simulink model "fixed_wing_sim"  (Simulink 8.7)
settings: Solver=ode4  StartTime=0.0  StopTime=T_sim  FixedStep=ts_sim  MaxStep=10e-3  RelTol=1e-3
InitFcn:
  | % Run the initialization script
  | clear all
  | aerosonde_uav_conf_model
StopFcn:
  | %show_result
  | print_results
values from neighbouring files (symbols this model uses):
  a = param(1)    [get_field.m]    (also in print_results.m = a*scale_fac/1e3; vector_field_parameters.m = 0.85)
  AilBnd = range_ail.*degrees2rad    [aerosonde_uav_conf_model.m]
  aileron_limits = [-20*pi/180;20*pi/180]    [aerosonde_uav_conf_model.m]
  AlphaBnd = range_alpha.*degrees2rad    [aerosonde_uav_conf_model.m]
  amp_theta = amp_theta*2    [vector_field_parameters.m]
  amp_theta_c = ((1/4)*[1 1 1]/6)*U_theta*tau_theta    [vector_field_parameters.m]
  amp_v_c = [1 1 1]*(tau_v*U_v)/6    [vector_field_parameters.m]
  amp_x = [5 5 5]    [vector_field_parameters.m]
  amp_y = [5 5 5]    [vector_field_parameters.m]
  amp_z = amp_z*2    [vector_field_parameters.m]
  amp_z_c = [1 1 1]*(tau_z*U_z)/6/2    [vector_field_parameters.m]
  b = param(2)    [get_field.m]    (also in print_results.m = b*scale_fac/1e3; vector_field_parameters.m = 0.08)
  BetaBnd = range_beta.*degrees2rad    [aerosonde_uav_conf_model.m]
  Bw = 2.8956    [aerosonde_uav_conf_model.m]
  c = param(3)    [get_field.m]    (also in vector_field_parameters.m = -0.13)
  CD_0 = 0.0434    [aerosonde_uav_conf_model.m]
  CD_ail = ones(length(AlphaBnd),1)*CD_aux_ail    [aerosonde_uav_conf_model.m]
  CD_alpha_beta = zeros(length(AlphaBnd),length(BetaBnd))    [aerosonde_uav_conf_model.m]
  CD_elev = ones(length(AlphaBnd),1)*CD_aux_elev    [aerosonde_uav_conf_model.m]
  CD_mind = 0.23    [aerosonde_uav_conf_model.m]
  CD_rud = ones(length(AlphaBnd),1)*CD_aux_rud    [aerosonde_uav_conf_model.m]
  CL_0 = 0.23    [aerosonde_uav_conf_model.m]
  Cl_ail = ones(length(AlphaBnd),1)*Cl_aux_ail    [aerosonde_uav_conf_model.m]
  CL_alpha_beta = CL_alpha*ones(1,length(BetaBnd))    [aerosonde_uav_conf_model.m]
  Cl_alpha_beta = ones(length(AlphaBnd),1)*Cl_beta    [aerosonde_uav_conf_model.m]
  CL_alphadot = 1.9724    [aerosonde_uav_conf_model.m]
  CL_elev = ones(length(AlphaBnd),1)*CL_aux_elev    [aerosonde_uav_conf_model.m]
  Cl_P = ones(length(AlphaBnd),1)*Cl_aux_P    [aerosonde_uav_conf_model.m]
  CL_Q = 7.9543*QBnd    [aerosonde_uav_conf_model.m]
  Cl_R = ones(length(AlphaBnd),1)*Cl_aux_R    [aerosonde_uav_conf_model.m]
  Cl_rud = ones(length(AlphaBnd),1)*Cl_aux_rud    [aerosonde_uav_conf_model.m]
  CLE_alphat = zeros(1,length(AlphaBnd))    [aerosonde_uav_conf_model.m]
  CLE_elev = 0    [aerosonde_uav_conf_model.m]
  Cm0 = 0.135    [aerosonde_uav_conf_model.m]
  Cm_alpha_beta = Cm_alpha*ones(1,length(BetaBnd))    [aerosonde_uav_conf_model.m]
  Cm_alphadot = -10.3796    [aerosonde_uav_conf_model.m]
  Cm_elev = ones(length(AlphaBnd),1)*Cm_aux_elev    [aerosonde_uav_conf_model.m]
  Cm_Q = -38.2067*QBnd    [aerosonde_uav_conf_model.m]
  Cn_ail = ones(length(AlphaBnd),1)*Cn_aux_ail    [aerosonde_uav_conf_model.m]
  Cn_alpha_beta = ones(length(AlphaBnd),1)*Cn_beta    [aerosonde_uav_conf_model.m]
  Cn_P = ones(length(AlphaBnd),1)*Cn_aux_P    [aerosonde_uav_conf_model.m]
  Cn_R = ones(length(AlphaBnd),1)*Cn_aux_R    [aerosonde_uav_conf_model.m]
  Cn_rud = ones(length(AlphaBnd),1)*Cn_aux_rud    [aerosonde_uav_conf_model.m]
  CT_save = CT_save.*10    [aerosonde_uav_conf_model.m]    (also in helice.mat = [0.115262 0.00375054783545 -0.00666475255621 -0.006665219028)
  curve = 1    [vector_field_parameters.m]
  Cw = 0.189941    [aerosonde_uav_conf_model.m]
  CY_ail = ones(length(AlphaBnd),1)*CY_aux_ail    [aerosonde_uav_conf_model.m]
  CY_alpha_beta = ones(length(AlphaBnd),1)*CY_beta    [aerosonde_uav_conf_model.m]
  CY_P = zeros(length(AlphaBnd),length(PBnd))    [aerosonde_uav_conf_model.m]
  CY_R = zeros(length(AlphaBnd),length(RBnd))    [aerosonde_uav_conf_model.m]
  CY_rud = ones(length(AlphaBnd),1)*CY_aux_rud    [aerosonde_uav_conf_model.m]
  d = param(4)    [get_field.m]    (also in vector_field_parameters.m = -0.04)
  D_hel = 0.15    [aerosonde_uav_conf_model.m]
  d_wash = 0    [aerosonde_uav_conf_model.m]
  delta_CD = 1    [aerosonde_uav_conf_model.m]
  delta_CL = 1    [aerosonde_uav_conf_model.m]
  delta_Cl = 1    [aerosonde_uav_conf_model.m]
  delta_Cm = 1    [aerosonde_uav_conf_model.m]
  delta_Cn = 1    [aerosonde_uav_conf_model.m]
  delta_CY = 1    [aerosonde_uav_conf_model.m]
  delta_FT = 1    [aerosonde_uav_conf_model.m]
  Delta_V_EH = [ 2 1.7365 1.2985 1.0890 1.0205]    [aerosonde_uav_conf_model.m]
  Delta_V_J = [ 0 0.4 0.7 1.4 2.1]    [aerosonde_uav_conf_model.m]
  elevator_limits = [-15*pi/180;15*pi/180]    [aerosonde_uav_conf_model.m]
  ElevBnd = range_elev.*degrees2rad    [aerosonde_uav_conf_model.m]
  F_T = 19    [aerosonde_uav_conf_model.m]
  f_theta = ([5 3 1]+rand(1,3))*0.05*2*pi/freq_divisor    [vector_field_parameters.m]
  f_theta_c = ([5 3 1]+rand(1,3))*0.05*2*pi/freq_divisor    [vector_field_parameters.m]
  f_v_c = ([4 2 0.5]+rand(1,3))*0.05*2*pi/freq_divisor    [vector_field_parameters.m]
  f_x = ([6 4 2]+rand(1,3))*0.05*2*pi/freq_divisor    [vector_field_parameters.m]
  f_y = ([6 4 2]+rand(1,3))*0.05*2*pi/freq_divisor    [vector_field_parameters.m]
  f_z = ([6 4 2]+rand(1,3))*0.05*2*pi/freq_divisor    [vector_field_parameters.m]
  f_z_c = ([4 2 0.5]+rand(1,3))*0.05*2*pi/freq_divisor    [vector_field_parameters.m]
  g1 = param(5)    [get_field.m]    (also in vector_field_parameters.m = 4)
  gain_G = param(6)    [get_field.m]    (also in vector_field_parameters.m = 2.5)
  gravity = 9.807    [aerosonde_uav_conf_model.m]
  H_0 = 200    [vector_field_parameters.m]
  Heq = 200    [aerosonde_uav_conf_model.m]    (also in vector_field_parameters.m)
  induced_drag = 1/(pi*AR*osw)    (= 0.0278403324809)    [aerosonde_uav_conf_model.m]
  isTrimming = 0    [aerosonde_uav_conf_model.m]
  J_save = J_save.*1.5    [aerosonde_uav_conf_model.m]    (also in helice.mat = [0 1.22229381539 1.27367709689 1.27367940534 1.27361400442 1)
  Jx = 0.7795    [aerosonde_uav_conf_model.m]
  Jxz = 0.1211    [aerosonde_uav_conf_model.m]
  Jy = 1.122    [aerosonde_uav_conf_model.m]
  Jz = 1.752    [aerosonde_uav_conf_model.m]
  KC_h = 0.28    [aerosonde_uav_conf_model.m]
  KC_phi = -1.18    [aerosonde_uav_conf_model.m]
  KC_psi = 0.03    [aerosonde_uav_conf_model.m]
  KC_r = -0.0073    [aerosonde_uav_conf_model.m]
  KC_theta = -1.1482    [aerosonde_uav_conf_model.m]
  KC_vt = 0.9948*1    (= 0.9948)    [aerosonde_uav_conf_model.m]
  KE = -0.1562    [aerosonde_uav_conf_model.m]
  Kp = 0.18    [vector_field_parameters.m]
  KR = 0.0130    (= 0.013)    [aerosonde_uav_conf_model.m]
  Ksad = param(3)    [get_field.m]    (also in print_results.m = Ksad*scale_fac/1e3; vector_field_parameters.m = 0)
  KT = 0.0792    [aerosonde_uav_conf_model.m]
  Kv = 1    [vector_field_parameters.m]
  LIM_CENTER = LIM_CENTER*scale_fac/1e3    [print_results.m]    (also in vector_field_parameters.m = 0.2)
  M = 8.5    [aerosonde_uav_conf_model.m]    (also in print_results.m = 0)
  motor_min = 0.1    [aerosonde_uav_conf_model.m]
  motor_rate = 1    [aerosonde_uav_conf_model.m]
  p_theta = rand(1,3)*2*pi    [vector_field_parameters.m]
  p_theta_c = rand(1,3)*2*pi    [vector_field_parameters.m]
  p_v_c = rand(1,3)*2*pi    [vector_field_parameters.m]
  p_x = rand(1,3)*2*pi    [vector_field_parameters.m]
  p_y = rand(1,3)*2*pi    [vector_field_parameters.m]
  p_z = rand(1,3)*2*pi    [vector_field_parameters.m]
  p_z_c = rand(1,3)*2*pi    [vector_field_parameters.m]
  PBnd = range_P.*degrees2rad    [aerosonde_uav_conf_model.m]
  perc_int_max = 0.8    [aerosonde_uav_conf_model.m]
  phi_max = 20*pi/180    (= 0.349065850399)    [aerosonde_uav_conf_model.m]
  phi_min = -20*pi/180    (= -0.349065850399)    [aerosonde_uav_conf_model.m]
  QBnd = range_Q.*degrees2rad    [aerosonde_uav_conf_model.m]
  r = sqrt(m)    [animation.m]    (also in print_results.m)
  r_aero_abc = r_aero_struct*[-1 0 0;0 1 0;0 0 -1]    [aerosonde_uav_conf_model.m]
  r_cg_abc = r_cg_struct*[-1 0 0;0 1 0;0 0 -1]    [aerosonde_uav_conf_model.m]
  r_motor_abc = r_motor_struct*[-1 0 0;0 1 0;0 0 -1]    [aerosonde_uav_conf_model.m]
  r_tail_abc = r_aero_struct*[-1 0 0;0 1 0;0 0 -1]    [aerosonde_uav_conf_model.m]
  RBnd = range_R.*degrees2rad    [aerosonde_uav_conf_model.m]
  rho = 0.1    [aerosonde_uav_conf_model.m]
  ... (+40 more)
undefined symbols (not defined in the file or in its folder): Earth, F, Light, MIL, WGS84
libraries: aerolibwind2 x2, aerolibtransform2 x2, aerolibfltsims x1, aerolibconvert2 x1, dspsigops x1
(part 1 of 3)
settings Model: Creator=torres  LastModifiedBy=adrianomcr  SimulationMode=accelerator
settings DataIOCC: SignalLoggingSaveFormat=ModelDataLogs  InspectSignalLogs=on
settings OptimizationCC: ExpressionDepthLimit=2147483647  EfficientMapNaN2IntZero=off
settings DebuggingCC: SolverPrmCheckMsg=warning  FcnCallInpInsideContextMsg=UseLocalSettings  UnconnectedInputMsg=none  UnconnectedOutputMsg=none  StateNameClashWarn=warning
settings HardwareCC: TargetBitPerLong=64  TargetBitPerPointer=64  TargetLongLongMode=on  TargetIntDivRoundTo=Zero  TargetEndianess=LittleEndian  TargetWordSize=64  TargetHWDeviceType=MATLAB Host  ProdEqTarget=off
settings SFSimCC: SimParseCustomCode=off
settings CodeAppCC: MaxIdLength=128
settings GRTTargetCC: GeneratePreprocessorConditionals=Use local settings  CombineOutputUpdateFcns=off  GRTInterface=on
settings ConfigComp: CovSFcnEnable=off

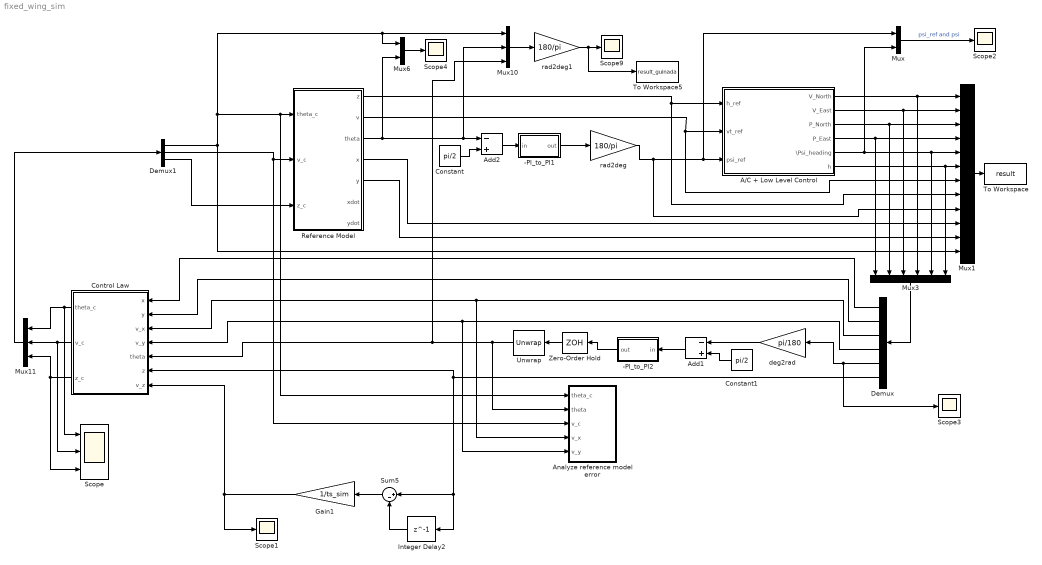
== system fixed_wing_sim ==
  -PI_to_PI1 : Subsystem
      mask Display: disp('-pi to pi')
  -PI_to_PI2 : Subsystem
      mask Display: disp('-pi to pi')
  "A/C + Low Level Control " : Subsystem
  Add1 : Sum  Inputs=-+
  Add2 : Sum  Inputs=-+
  Analyze reference model error : Subsystem
  Constant : Constant  Value=pi/2
  Constant1 : Constant  Value=pi/2
  Control Law : Subsystem
  Demux : Demux  Outputs=6
  Demux1 : Demux  Outputs=3
  Gain1 : Gain  Gain=1/ts_sim
  Integer Delay2 : Delay  DelayLength=1  InitialCondition=H_0  InputProcessing=Inherited
  Mux : Mux  Inputs=2
  Mux1 : Mux  Inputs=12
  Mux10 : Mux  Inputs=3
  Mux11 : Mux  Inputs=3
  Mux3 : Mux  Inputs=6
  Mux6 : Mux  Inputs=2
  Reference Model : Subsystem
  Scope : Scope  NumInputPorts=3
  Scope{1..4,9} (5 alike) : Scope
  Sum5 : Sum  Inputs=|+-
  To Workspace : ToWorkspace  VariableName=result  SaveFormat=Structure With Time  SampleTime=-1
  To Workspace5 : ToWorkspace  VariableName=result_guinada  SaveFormat=Structure With Time  SampleTime=-1
  Unwrap : dspsigops/Unwrap  tol=pi  InputProcessing=Inherited (this choice will be removed - see release notes)  running=off
  Zero-Order Hold : ZeroOrderHold  SampleTime=ts_sim
  deg2rad : Gain  Gain=pi/180
  rad2deg : Gain  Gain=180/pi
  rad2deg1 : Gain  Gain=180/pi
  wires:
  Add2/1 -> -PI_to_PI1/1(in)
  "A/C + Low Level Control "/5(\Psi_heading) -> Mux1/5, Mux3/5, Mux/2
  Reference Model/2(v) -> "A/C + Low Level Control "/2(vt_ref), Mux1/7
  Mux/1 -> Scope2/1  "psi_ref and psi"
  Reference Model/1(z) -> Mux1/8, "A/C + Low Level Control "/1(h_ref)
  -PI_to_PI1/1(out) -> rad2deg/1
  rad2deg/1 -> Mux/1, "A/C + Low Level Control "/3(psi_ref), Mux1/9
  Mux1/1 -> To Workspace/1
  "A/C + Low Level Control "/1(V_North) -> Mux1/1, Mux3/4
  "A/C + Low Level Control "/2(V_East) -> Mux1/2, Mux3/3
  "A/C + Low Level Control "/3(P_North) -> Mux1/3, Mux3/2
  "A/C + Low Level Control "/4(P_East) -> Mux1/4, Mux3/1
  "A/C + Low Level Control "/6(h) -> Mux3/6, Mux1/6
  Add1/1 -> -PI_to_PI2/1(in)
  Constant1/1 -> Add1/2
  deg2rad/1 -> Add1/1
  Demux/3 -> Analyze reference model error/4(v_x), Control Law/3(v_x)
  Mux3/1 -> Demux/1
  Mux6/1 -> Scope4/1
  Demux/5 -> Scope3/1, deg2rad/1
  Demux/1 -> Control Law/1(x)
  Demux/2 -> Control Law/2(y)
  Zero-Order Hold/1 -> Unwrap/1
  -PI_to_PI2/1(out) -> Zero-Order Hold/1
  Mux10/1 -> rad2deg1/1
  Reference Model/3(theta) -> Mux6/2, Mux10/2, Add2/1
  Mux11/1 -> Demux1/1
  Demux1/2 -> Analyze reference model error/3(v_c), Reference Model/2(v_c)
  Demux1/1 -> Mux1/12, Analyze reference model error/1(theta_c), Reference Model/1(theta_c), Mux10/1, Mux6/1
  Constant/1 -> Add2/2
  rad2deg1/1 -> To Workspace5/1, Scope9/1
  Demux/4 -> Analyze reference model error/5(v_y), Control Law/4(v_y)
  Reference Model/4(x) -> Mux1/10
  Reference Model/5(y) -> Mux1/11
  Demux1/3 -> Reference Model/3(z_c)
  Demux/6 -> Integer Delay2/1, Sum5/1, Control Law/6(z)
  Sum5/1 -> Gain1/1
  Gain1/1 -> Scope1/1, Control Law/7(v_z)
  Integer Delay2/1 -> Sum5/2
  Control Law/1(theta_c) -> Scope/1, Mux11/1
  Control Law/2(v_c) -> Scope/2, Mux11/2
  Control Law/3(z_c) -> Mux11/3, Scope/3
  Unwrap/1 -> Analyze reference model error/2(theta), Control Law/5(theta), Mux10/3

== system fixed_wing_sim/-PI_to_PI1 ==
  in : Inport
  Constant : Constant  Value=pi
  Fcn : Fcn  Expr=atan2(sin(u),cos(u))
  Gain : Gain  Gain=2
  Math Function : Math  Operator=mod  SaturateOnIntegerOverflow=on
  Sum : Sum  Inputs=|++
  Sum1 : Sum  Inputs=|+-
  out : Outport
  wires:
  Constant/1 -> Sum/2, Gain/1, Sum1/2
  Sum/1 -> Math Function/1
  Gain/1 -> Math Function/2
  Math Function/1 -> Sum1/1
  in/1 -> Fcn/1
  Fcn/1 -> out/1

== system fixed_wing_sim/-PI_to_PI2 ==
  in : Inport
  Constant : Constant  Value=pi
  Fcn : Fcn  Expr=atan2(sin(u),cos(u))
  Gain : Gain  Gain=2
  Math Function : Math  Operator=mod  SaturateOnIntegerOverflow=on
  Sum : Sum  Inputs=|++
  Sum1 : Sum  Inputs=|+-
  out : Outport
  wires:
  Constant/1 -> Sum/2, Gain/1, Sum1/2
  Sum/1 -> Math Function/1
  Gain/1 -> Math Function/2
  Math Function/1 -> Sum1/1
  in/1 -> Fcn/1
  Fcn/1 -> out/1

== system fixed_wing_sim/A/C + Low Level Control  ==
  h_ref : Inport
  vt_ref : Inport  Port=2
  psi_ref : Inport  Port=3
  -180_to_180 : Subsystem
      mask Display: disp('-180 to +180')
  Abs : Abs
  Add1 : Sum  Inputs=+-
  Add4 : Sum  Inputs=-+
  Gain : Gain  Gain=KE
  Gain1 : Gain  Gain=KT
  PID h : Subsystem
  PID psi (modified) : Subsystem
  UAV Internal Closed Loops : Subsystem
  V_North : Outport
  V_East : Outport  Port=2
  P_North : Outport  Port=3
  P_East : Outport  Port=4
  \Psi_heading : Outport  Port=5
  h : Outport  Port=6
  wires:
  PID h/1(theta_ref) -> UAV Internal Closed Loops/1(ref_theta)
  Add4/1 -> PID h/1(erro), Gain1/1
  PID psi (modified)/1(phi_ref) -> Abs/1, UAV Internal Closed Loops/2(ref_phi)
  Gain1/1 -> UAV Internal Closed Loops/3(uk_thro)
  Add1/1 -> -180_to_180/1(in)
  Gain/1 -> UAV Internal Closed Loops/4(uk_elev)
  UAV Internal Closed Loops/4(\Psi_heading) -> Add1/2, \Psi_heading/1
  Abs/1 -> Gain/1
  UAV Internal Closed Loops/3(h) -> Add4/1, h/1
  h_ref/1 -> Add4/2
  psi_ref/1 -> Add1/1
  vt_ref/1 -> UAV Internal Closed Loops/5(ref_vt)
  UAV Internal Closed Loops/1(V_North) -> V_North/1
  UAV Internal Closed Loops/5(P_North) -> P_North/1
  UAV Internal Closed Loops/6(P_East) -> P_East/1
  UAV Internal Closed Loops/2(V_East) -> V_East/1
  -180_to_180/1(out) -> PID psi (modified)/1(erro)

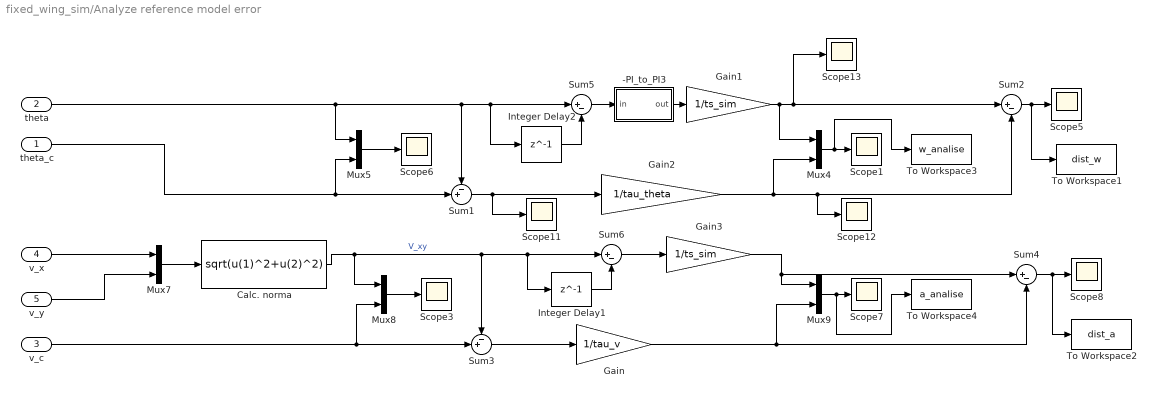
== system fixed_wing_sim/Analyze reference model error ==
  theta_c : Inport
  theta : Inport  Port=2
  v_c : Inport  Port=3
  v_x : Inport  Port=4
  v_y : Inport  Port=5
  -PI_to_PI3 : Subsystem
      mask Display: disp('-pi to pi')
  Calc. norma : Fcn  Expr=sqrt(u(1)^2+u(2)^2)
  Gain : Gain  Gain=1/tau_v
  Gain1 : Gain  Gain=1/ts_sim
  Gain2 : Gain  Gain=1/tau_theta
  Gain3 : Gain  Gain=1/ts_sim
  Integer Delay1 : Delay  DelayLength=1  InitialCondition=Veq  InputProcessing=Inherited
  Integer Delay2 : Delay  DelayLength=1  InitialCondition=theta_0  InputProcessing=Inherited
  Mux{4..5,7..9} (5 alike) : Mux  Inputs=2
  Scope{1,3,5..8,11..13} (9 alike) : Scope
  Sum1 : Sum  Inputs=-+|
  Sum{2,4..6} (4 alike) : Sum  Inputs=|+-
  Sum3 : Sum  Inputs=-+|
  To Workspace1 : ToWorkspace  VariableName=dist_w  SaveFormat=Structure With Time  SampleTime=-1
  To Workspace2 : ToWorkspace  VariableName=dist_a  SaveFormat=Structure With Time  SampleTime=-1
  To Workspace3 : ToWorkspace  VariableName=w_analise  SaveFormat=Structure With Time  SampleTime=-1
  To Workspace4 : ToWorkspace  VariableName=a_analise  SaveFormat=Structure With Time  SampleTime=-1
  wires:
  Sum2/1 -> To Workspace1/1, Scope5/1
  Mux5/1 -> Scope6/1
  Gain2/1 -> Mux4/2, Scope12/1, Sum2/2
  Calc. norma/1 -> Mux8/1, Sum3/1, Integer Delay1/1, Sum6/1  "V_xy"
  Mux8/1 -> Scope3/1
  Sum3/1 -> Gain/1
  Mux9/1 -> To Workspace4/1, Scope7/1
  Gain/1 -> Sum4/2, Mux9/2
  Sum4/1 -> To Workspace2/1, Scope8/1
  Integer Delay2/1 -> Sum5/2
  Gain1/1 -> Scope13/1, Sum2/1, Mux4/1
  Mux4/1 -> To Workspace3/1, Scope1/1
  Integer Delay1/1 -> Sum6/2
  Sum6/1 -> Gain3/1
  Gain3/1 -> Sum4/1, Mux9/1
  Sum1/1 -> Scope11/1, Gain2/1
  Sum5/1 -> -PI_to_PI3/1(in)
  -PI_to_PI3/1(out) -> Gain1/1
  Mux7/1 -> Calc. norma/1
  v_x/1 -> Mux7/1
  v_y/1 -> Mux7/2
  v_c/1 -> Sum3/2, Mux8/2
  theta_c/1 -> Mux5/2, Sum1/2
  theta/1 -> Mux5/1, Integer Delay2/1, Sum5/1, Sum1/1

== system fixed_wing_sim/Control Law ==
  x : Inport
  y : Inport  Port=2
  v_x : Inport  Port=3
  v_y : Inport  Port=4
  theta : Inport  Port=5
  z : Inport  Port=6
  v_z : Inport  Port=7
  Actuation Error : Subsystem
  Control law : MATLAB Function  TreatAsAtomicUnit=on
  Demux : Demux  Outputs=9
  Measurement Error : Subsystem
  Mux14 : Mux  Inputs=2
  Potental functions : Scope  NumInputPorts=2
  Potental functions1 : Scope  NumInputPorts=9
  Sum{,1..2,5} (4 alike) : Sum  Inputs=|++
  Sum3 : Sum  Inputs=++|
  Sum4 : Sum  Inputs=++|
  Sum6 : Sum  Inputs=++|
  To Workspace6 : ToWorkspace  VariableName=PotFncs  SaveFormat=Structure With Time  SampleTime=-1
  theta_c : Outport
  v_c : Outport  Port=2
  z_c : Outport  Port=3
  wires:
  v_x/1 -> Control law/3(xd)
  v_y/1 -> Control law/4(yd)
  Mux14/1 -> To Workspace6/1
  Control law/4(V_theta) -> Potental functions/1, Mux14/1
  Control law/5(V_fld) -> Potental functions/2, Mux14/2
  Sum/1 -> Control law/1(x)
  x/1 -> Sum/1
  Measurement Error/2(Noise_x) -> Sum/2
  Sum1/1 -> Control law/2(y)
  y/1 -> Sum1/1
  Measurement Error/3(Noise_y) -> Sum1/2
  Sum2/1 -> Control law/5(theta)
  Control law/1(theta_c) -> Sum3/2
  Sum3/1 -> theta_c/1
  Sum4/1 -> v_c/1
  Control law/2(v_c) -> Sum4/2
  Actuation Error/2(Noise_v_c) -> Sum4/1
  Actuation Error/1(Noise_theta_c) -> Sum3/1
  theta/1 -> Sum2/1
  Measurement Error/1(Noise_theta) -> Sum2/2
  v_z/1 -> Control law/7(zd)
  Sum5/1 -> Control law/6(z)
  z/1 -> Sum5/1
  Measurement Error/4(Noise_z) -> Sum5/2
  Sum6/1 -> z_c/1
  Control law/3(z_c) -> Sum6/2
  Actuation Error/3(Noise_z_c) -> Sum6/1
  Control law/6(teste) -> Demux/1
  Demux/1 -> Potental functions1/1
  Demux/2 -> Potental functions1/2
  Demux/9 -> Potental functions1/9
  Demux/8 -> Potental functions1/8
  Demux/7 -> Potental functions1/7
  Demux/6 -> Potental functions1/6
  Demux/5 -> Potental functions1/5
  Demux/4 -> Potental functions1/4
  Demux/3 -> Potental functions1/3

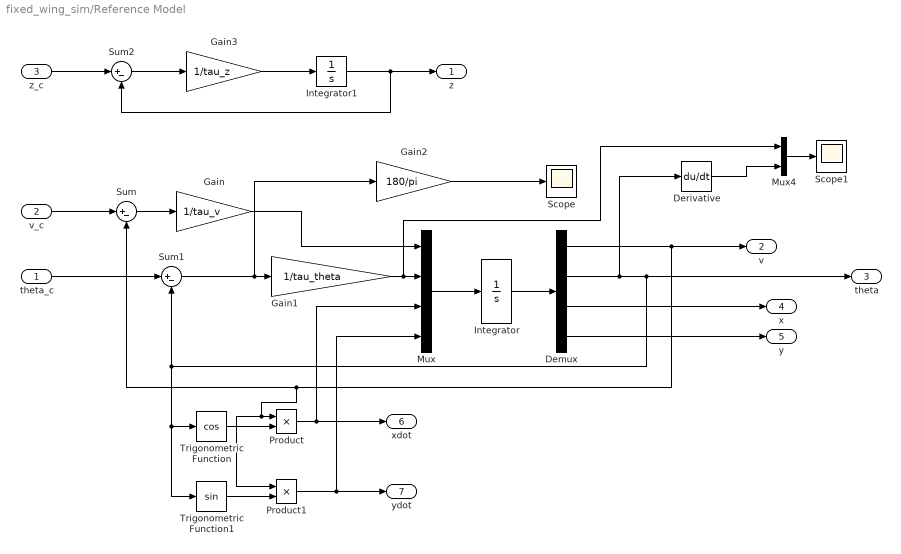
== system fixed_wing_sim/Reference Model ==
  theta_c : Inport
  v_c : Inport  Port=2
  z_c : Inport  Port=3
  Demux : Demux
  Derivative : Derivative
  Gain : Gain  Gain=1/tau_v
  Gain1 : Gain  Gain=1/tau_theta
  Gain2 : Gain  Gain=180/pi
  Gain3 : Gain  Gain=1/tau_z
  Integrator : Integrator  InitialCondition=x0_refmodel
  Integrator1 : Integrator  InitialCondition=H_0
  Mux : Mux
  Mux4 : Mux  Inputs=2
  Product : Product  RndMeth=Zero
  Product1 : Product  RndMeth=Zero
  Scope : Scope
  Scope1 : Scope
  Sum : Sum  Inputs=|+-
  Sum1 : Sum  Inputs=|+-
  Sum2 : Sum  Inputs=|+-
  Trigonometric Function : Trigonometry  Operator=cos
  Trigonometric Function1 : Trigonometry
  z : Outport
  v : Outport  Port=2
  theta : Outport  Port=3
  x : Outport  Port=4
  y : Outport  Port=5
  xdot : Outport  Port=6
  ydot : Outport  Port=7
  wires:
  v_c/1 -> Sum/1
  Sum/1 -> Gain/1
  Gain/1 -> Mux/1
  Sum1/1 -> Gain1/1, Gain2/1
  Gain1/1 -> Mux4/1, Mux/2
  theta_c/1 -> Sum1/1
  Mux/1 -> Integrator/1
  Integrator/1 -> Demux/1
  Demux/1 -> v/1, Product1/1, Product/1, Sum/2
  Demux/2 -> Derivative/1, theta/1, Trigonometric Function/1, Trigonometric Function1/1, Sum1/2
  Trigonometric Function/1 -> Product/2
  Trigonometric Function1/1 -> Product1/2
  Product/1 -> Mux/3, xdot/1
  Product1/1 -> Mux/4, ydot/1
  Demux/3 -> x/1
  Demux/4 -> y/1
  Gain2/1 -> Scope/1
  Mux4/1 -> Scope1/1
  Derivative/1 -> Mux4/2
  z_c/1 -> Sum2/1
  Sum2/1 -> Gain3/1
  Gain3/1 -> Integrator1/1
  Integrator1/1 -> Sum2/2, z/1

== system fixed_wing_sim/A/C + Low Level Control /-180_to_180 ==
  in : Inport
  Constant : Constant  Value=pi
  Gain : Gain  Gain=2
  Math Function : Math  Operator=mod  SaturateOnIntegerOverflow=on
  Sum : Sum  Inputs=|++
  Sum1 : Sum  Inputs=|+-
  deg2rad : Gain  Gain=pi/180
  rad2deg : Gain  Gain=180/pi
  out : Outport
  wires:
  Constant/1 -> Sum/2, Gain/1, Sum1/2
  in/1 -> deg2rad/1
  Sum/1 -> Math Function/1
  Gain/1 -> Math Function/2
  Math Function/1 -> Sum1/1
  Sum1/1 -> rad2deg/1
  rad2deg/1 -> out/1
  deg2rad/1 -> Sum/1

== system fixed_wing_sim/A/C + Low Level Control /PID h ==
  erro : Inport
  Add : Sum  Inputs=+-++
  Constant : Constant  Value=TI_h
  Divide : Product  Inputs=*/
  Gain : Gain  Gain=KC_h
  Gain1 : Gain
  Gain2 : Gain  Gain=1/rho
  Integrator : Integrator  InitialCondition=x0_uav(5)  LimitOutput=on  UpperSaturationLimit=perc_int_max*theta_max  LowerSaturationLimit=perc_int_max*theta_min
  Rate Limiter1 : RateLimiter  RisingSlewLimit=theta_rate  FallingSlewLimit=-theta_rate
  Saturation1 : Saturate  UpperLimit=theta_max  LowerLimit=theta_min
  Transfer Fcn : TransferFcn  Numerator=[1/rho]  Denominator=[rho*TD_h 1]
  theta_ref : Outport
  wires:
  Add/1 -> Rate Limiter1/1
  Transfer Fcn/1 -> Add/2
  Integrator/1 -> Add/4
  Divide/1 -> Integrator/1
  Constant/1 -> Divide/2
  Gain1/1 -> Add/1
  Gain2/1 -> Add/3
  erro/1 -> Gain/1
  Gain/1 -> Gain1/1, Transfer Fcn/1, Gain2/1, Divide/1
  Rate Limiter1/1 -> Saturation1/1
  Saturation1/1 -> theta_ref/1

== system fixed_wing_sim/A/C + Low Level Control /PID psi (modified) ==
  erro : Inport
  Add : Sum  Inputs=+-++
  Constant : Constant  Value=TI_psi
  Divide : Product  Inputs=*/
  Gain : Gain  Gain=KC_psi
  Gain1 : Gain
  Gain2 : Gain  Gain=1/rho
  Integrator : Integrator  LimitOutput=on  UpperSaturationLimit=phi_max  LowerSaturationLimit=phi_min
  Rate Limiter2 : RateLimiter  RisingSlewLimit=roll_rate  FallingSlewLimit=-roll_rate
  Saturation2 : Saturate  UpperLimit=phi_max  LowerLimit=phi_min
  Transfer Fcn : TransferFcn  Numerator=[1/rho]  Denominator=[rho*TD_psi 1]
  phi_ref : Outport
  wires:
  Transfer Fcn/1 -> Add/2
  Gain1/1 -> Add/1
  Gain2/1 -> Add/3
  erro/1 -> Gain/1
  Gain/1 -> Gain1/1, Transfer Fcn/1, Gain2/1, Divide/1
  Rate Limiter2/1 -> Saturation2/1
  Saturation2/1 -> phi_ref/1
  Add/1 -> Rate Limiter2/1
  Integrator/1 -> Add/4
  Divide/1 -> Integrator/1
  Constant/1 -> Divide/2

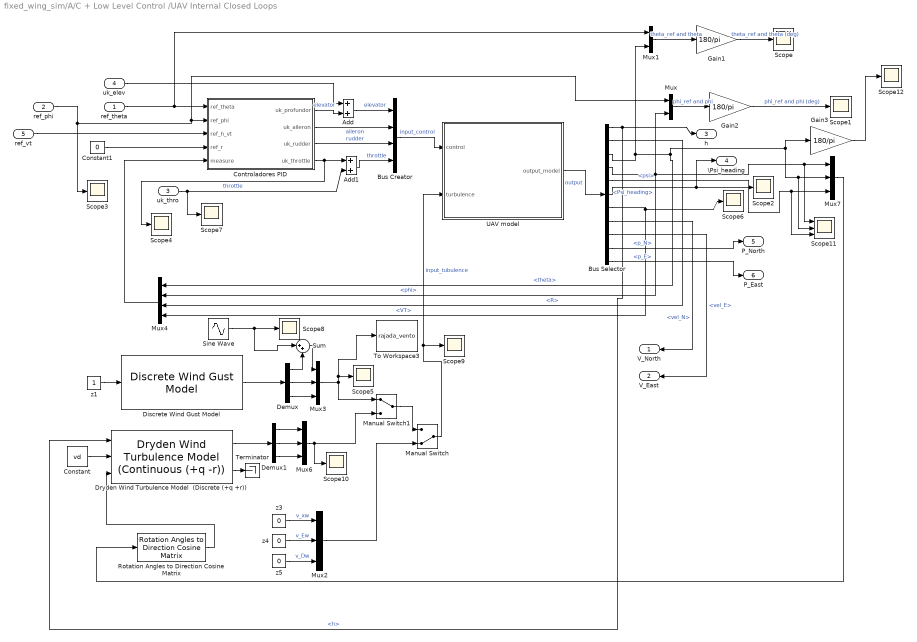
== system fixed_wing_sim/A/C + Low Level Control /UAV Internal Closed Loops ==
  ref_theta : Inport
  ref_phi : Inport  Port=2
  uk_thro : Inport  Port=3
  uk_elev : Inport  Port=4
  ref_vt : Inport  Port=5
  Add : Sum
  Add1 : Sum
  Bus Creator : BusCreator  Inputs=4
  Bus Selector : BusSelector  OutputSignals=h,R,theta,phi,psi,Psi_heading,VT,vel_N,vel_E,p_N,p_E
  Constant : Constant  Value=vd
  Constant1 : Constant  Value=0
  Controladores PID : Subsystem
  Demux : Demux  Outputs=3
  Demux1 : Demux  Outputs=3
  Discrete Wind Gust Model : aerolibwind2/Discrete Wind Gust Model  units=Metric (MKS)  Gx=on  Gy=on  Gz=on  t_0=0  d_m=[20 20 20]  v_m=[5.75 0 0]
  Dryden Wind Turbulence Model  (Discrete (+q +r)) : aerolibwind2/Dryden Wind Turbulence Model  (Continuous (+q -r))  units=Metric (MKS)  spec=MIL-F-8785C  model=Continuous Dryden (+q +r)  W20=1  Wdeg=0  TurbProb=10^-2 - Light  L_high=533.4  Wingspan=Bw  ts=ts_sim  Seed=[23341 23342 23343 23344]  T_on=on
  Gain1 : Gain  Gain=180/pi
  Gain2 : Gain  Gain=180/pi
  Gain3 : Gain  Gain=180/pi
  Manual Switch : ManualSwitch  CurrentSetting=0
  Manual Switch1 : ManualSwitch
  Mux : Mux  Inputs=2
  Mux1 : Mux  Inputs=2
  Mux{2..3,6..7} (4 alike) : Mux  Inputs=3
  Mux4 : Mux
  Rotation Angles to Direction Cosine Matrix : aerolibtransform2/Rotation Angles to Direction Cosine Matrix  rotationOrder=ZYX
  Scope{,1..10,12} (12 alike) : Scope
  Scope11 : Scope  NumInputPorts=3
  Sine Wave : Sin  Amplitude=2  Frequency=0.1  SampleTime=0
  Sum : Sum  Inputs=|++
  Terminator : Terminator
  To Workspace3 : ToWorkspace  VariableName=rajada_vento  SaveFormat=Structure With Time  SampleTime=-1
  UAV model : Subsystem
      mask Display: image(imread('Figures/rascal.jpg'))
  z1 : Constant
  z3 : Constant  Value=0
  z4 : Constant  Value=0
  z5 : Constant  Value=0
  V_North : Outport
  V_East : Outport  Port=2
  h : Outport  Port=3
  \Psi_heading : Outport  Port=4
  P_North : Outport  Port=5
  P_East : Outport  Port=6
  wires:
  Controladores PID/3(uk_rudder) -> Bus Creator/3  "rudder"
  UAV model/1(output_model) -> Bus Selector/1  "output"
  Bus Creator/1 -> UAV model/1(control)  "input_control"
  Manual Switch/1 -> UAV model/2(turbulence), Scope9/1  "input_tubulence"
  z4/1 -> Mux2/2  "v_Ew"
  z5/1 -> Mux2/3  "v_Dw"
  Mux4/1 -> Controladores PID/5(measure)
  Bus Selector/7 -> Scope6/1, Mux4/4  "<VT>"
  Controladores PID/2(uk_aileron) -> Bus Creator/2  "aileron"
  Bus Selector/2 -> Mux4/3  "<R>"
  ref_theta/1 -> Controladores PID/1(ref_theta), Mux1/1
  ref_phi/1 -> Controladores PID/2(ref_phi), Mux/1, Scope3/1
  Constant1/1 -> Controladores PID/4(ref_r)
  Controladores PID/4(uk_throttle) -> Scope4/1, Add1/1  "throttle"
  Add1/1 -> Bus Creator/4  "throttle"
  uk_thro/1 -> Scope7/1, Add1/2
  Controladores PID/1(uk_profundor) -> Add/2  "elevator"
  Add/1 -> Bus Creator/1  "elevator"
  uk_elev/1 -> Add/1
  Mux1/1 -> Gain1/1  "theta_ref and theta"
  Mux/1 -> Gain2/1  "phi_ref and phi"
  ref_vt/1 -> Controladores PID/3(ref_h_vt)
  Bus Selector/8 -> V_North/1  "<vel_N>"
  Bus Selector/9 -> V_East/1  "<vel_E>"
  Bus Selector/10 -> P_North/1  "<p_N>"
  Bus Selector/11 -> P_East/1  "<p_E>"
  Bus Selector/1 -> Dryden Wind Turbulence Model  (Discrete (+q +r))/1, h/1  "<h>"
  Bus Selector/6 -> Scope2/1, \Psi_heading/1  "<Psi_heading>"
  Bus Selector/4 -> Mux4/2, Scope11/1, Mux7/1, Mux/2  "<phi>"
  Bus Selector/3 -> Mux4/1, Scope11/2, Mux7/2, Gain3/1, Mux1/2  "<theta>"
  Gain1/1 -> Scope/1  "theta_ref and theta (deg)"
  Gain2/1 -> Scope1/1  "phi_ref and phi (deg)"
  z1/1 -> Discrete Wind Gust Model/1
  z3/1 -> Mux2/1  "v_xw"
  Mux2/1 -> Manual Switch/2
  Discrete Wind Gust Model/1 -> Demux/1
  Demux/2 -> Mux3/2
  Demux/3 -> Mux3/3
  Mux3/1 -> To Workspace3/1, Scope5/1, Manual Switch1/1
  Demux1/2 -> Mux6/2
  Demux1/3 -> Mux6/3
  Demux1/1 -> Mux6/1
  Mux6/1 -> Manual Switch1/2, Scope10/1
  Dryden Wind Turbulence Model  (Discrete (+q +r))/2 -> Terminator/1
  Rotation Angles to Direction Cosine Matrix/1 -> Dryden Wind Turbulence Model  (Discrete (+q +r))/3
  Mux7/1 -> Rotation Angles to Direction Cosine Matrix/1
  Bus Selector/5 -> Scope11/3, Mux7/3  "<psi>"
  Constant/1 -> Dryden Wind Turbulence Model  (Discrete (+q +r))/2
  Manual Switch1/1 -> Manual Switch/1
  Dryden Wind Turbulence Model  (Discrete (+q +r))/1 -> Demux1/1
  Sine Wave/1 -> Scope8/1, Sum/1
  Demux/1 -> Sum/2
  Sum/1 -> Mux3/1
  Gain3/1 -> Scope12/1

== system fixed_wing_sim/Analyze reference model error/-PI_to_PI3 ==
  in : Inport
  Constant : Constant  Value=pi
  Fcn : Fcn  Expr=atan2(sin(u),cos(u))
  Gain : Gain  Gain=2
  Math Function : Math  Operator=mod  SaturateOnIntegerOverflow=on
  Sum : Sum  Inputs=|++
  Sum1 : Sum  Inputs=|+-
  out : Outport
  wires:
  Constant/1 -> Sum/2, Gain/1, Sum1/2
  Sum/1 -> Math Function/1
  Gain/1 -> Math Function/2
  Math Function/1 -> Sum1/1
  in/1 -> Fcn/1
  Fcn/1 -> out/1

== system fixed_wing_sim/Control Law/Actuation Error ==
  note: Disturbance in the theta_c control signal
  note: Disturbance in the v_c control signal
  note: Disturbance in the z_c control signal
  Constant : Constant  Value=0.0001
  Constant1 : Constant  Value=0.0001
  Constant2 : Constant  Value=0.0001
  Demux : Demux  Outputs=3
  Gain : Gain
  Gain1 : Gain  Gain=0.8
  Gain2 : Gain  Gain=0.001
  Manual Switch Noise : ManualSwitch
  Mux1 : Mux  Inputs=3
  Mux14 : Mux  Inputs=3
  Scope : Scope  NumInputPorts=3
  Sine Wave : Sin  Amplitude=amp_theta_c(1)  Frequency=f_theta_c(1)  Phase=p_theta_c(1)  SampleTime=0
  Sine Wave1 : Sin  Amplitude=amp_theta_c(2)  Frequency=f_theta_c(2)  Phase=p_theta_c(2)  SampleTime=0
  Sine Wave2 : Sin  Amplitude=amp_theta_c(3)  Frequency=f_theta_c(3)  Phase=p_theta_c(3)  SampleTime=0
  Sine Wave3 : Sin  Amplitude=amp_v_c(1)  Frequency=f_v_c(1)  Phase=p_v_c(1)  SampleTime=0
  Sine Wave4 : Sin  Amplitude=amp_v_c(2)  Frequency=f_v_c(2)  Phase=p_v_c(2)  SampleTime=0
  Sine Wave5 : Sin  Amplitude=amp_v_c(3)  Frequency=f_v_c(3)  Phase=p_v_c(3)  SampleTime=0
  Sine Wave6 : Sin  Amplitude=amp_z_c(1)  Frequency=f_z_c(1)  Phase=p_z_c(1)  SampleTime=0
  Sine Wave7 : Sin  Amplitude=amp_z_c(2)  Frequency=f_z_c(2)  Phase=p_z_c(2)  SampleTime=0
  Sine Wave8 : Sin  Amplitude=amp_z_c(3)  Frequency=f_z_c(3)  Phase=p_z_c(3)  SampleTime=0
  Sum : Sum  Inputs=+++
  Sum1 : Sum  Inputs=+++
  Sum2 : Sum  Inputs=+++
  Noise_theta_c : Outport
  Noise_v_c : Outport  Port=2
  Noise_z_c : Outport  Port=3
  wires:
  Sine Wave1/1 -> Sum/2
  Sine Wave/1 -> Sum/1
  Sine Wave2/1 -> Sum/3
  Sine Wave4/1 -> Sum1/2
  Sine Wave3/1 -> Sum1/1
  Sine Wave5/1 -> Sum1/3
  Sum/1 -> Scope/1, Mux14/1  "Noise theta_c"
  Sum1/1 -> Gain/1
  Constant1/1 -> Mux1/2
  Constant/1 -> Mux1/1
  Mux14/1 -> Manual Switch Noise/1
  Mux1/1 -> Gain2/1
  Manual Switch Noise/1 -> Gain1/1
  Demux/2 -> Noise_v_c/1
  Demux/1 -> Noise_theta_c/1
  Gain/1 -> Scope/2, Mux14/2  "Noise v_c"
  Sine Wave7/1 -> Sum2/2
  Sine Wave6/1 -> Sum2/1
  Sine Wave8/1 -> Sum2/3
  Constant2/1 -> Mux1/3
  Sum2/1 -> Scope/3, Mux14/3  "Noise z_c"
  Demux/3 -> Noise_z_c/1
  Gain1/1 -> Demux/1
  Gain2/1 -> Manual Switch Noise/2

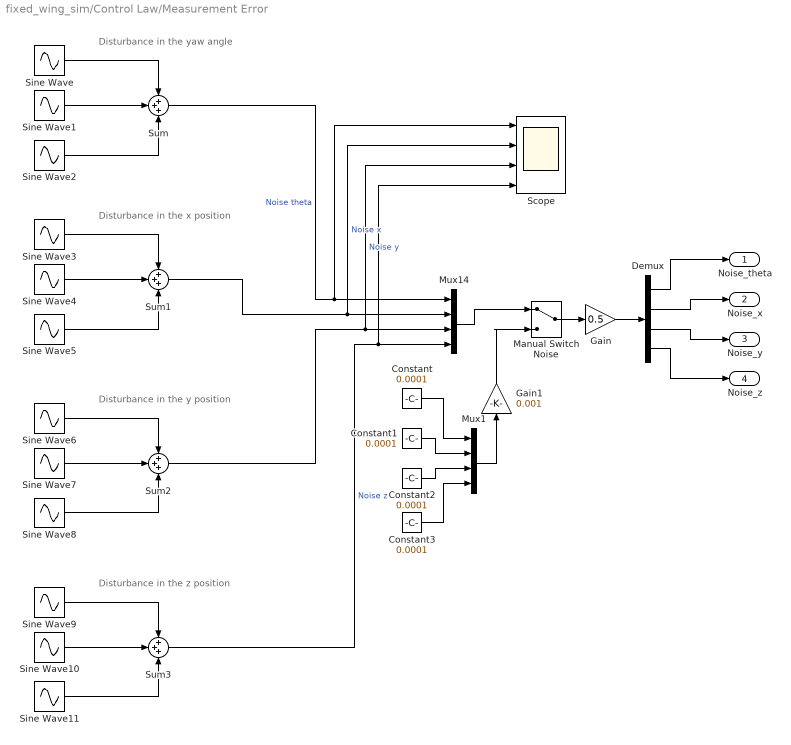
== system fixed_wing_sim/Control Law/Measurement Error ==
  note: Disturbance in the yaw angle
  note: Disturbance in the x position
  note: Disturbance in the y position
  note: Disturbance in the z position
  Constant{,1..3} (4 alike) : Constant  Value=0.0001
  Demux : Demux
  Gain : Gain  Gain=0.5
  Gain1 : Gain  Gain=0.001
  Manual Switch Noise : ManualSwitch
  Mux1 : Mux
  Mux14 : Mux
  Scope : Scope  NumInputPorts=4
  Sine Wave : Sin  Amplitude=amp_theta(1)  Frequency=f_theta(1)  Phase=p_theta(1)  SampleTime=0
  Sine Wave1 : Sin  Amplitude=amp_theta(2)  Frequency=f_theta(2)  Phase=p_theta(2)  SampleTime=0
  Sine Wave10 : Sin  Amplitude=amp_z(2)  Frequency=f_z(2)  Phase=p_z(2)  SampleTime=0
  Sine Wave11 : Sin  Amplitude=amp_z(3)  Frequency=f_z(3)  Phase=p_z(3)  SampleTime=0
  Sine Wave2 : Sin  Amplitude=amp_theta(3)  Frequency=f_theta(3)  Phase=p_theta(3)  SampleTime=0
  Sine Wave3 : Sin  Amplitude=amp_x(1)  Frequency=f_x(1)  Phase=p_x(1)  SampleTime=0
  Sine Wave4 : Sin  Amplitude=amp_x(2)  Frequency=f_x(2)  Phase=p_x(2)  SampleTime=0
  Sine Wave5 : Sin  Amplitude=amp_x(3)  Frequency=f_x(3)  Phase=p_x(3)  SampleTime=0
  Sine Wave6 : Sin  Amplitude=amp_y(1)  Frequency=f_y(1)  Phase=p_y(1)  SampleTime=0
  Sine Wave7 : Sin  Amplitude=amp_y(2)  Frequency=f_y(2)  Phase=p_y(2)  SampleTime=0
  Sine Wave8 : Sin  Amplitude=amp_y(3)  Frequency=f_y(3)  Phase=p_y(3)  SampleTime=0
  Sine Wave9 : Sin  Amplitude=amp_z(1)  Frequency=f_z(1)  Phase=p_z(1)  SampleTime=0
  Sum{,1..3} (4 alike) : Sum  Inputs=+++
  Noise_theta : Outport
  Noise_x : Outport  Port=2
  Noise_y : Outport  Port=3
  Noise_z : Outport  Port=4
  wires:
  Sine Wave1/1 -> Sum/2
  Sine Wave/1 -> Sum/1
  Sine Wave2/1 -> Sum/3
  Sine Wave4/1 -> Sum1/2
  Sine Wave3/1 -> Sum1/1
  Sine Wave5/1 -> Sum1/3
  Sine Wave7/1 -> Sum2/2
  Sine Wave6/1 -> Sum2/1
  Sine Wave8/1 -> Sum2/3
  Sum/1 -> Scope/1, Mux14/1  "Noise theta"
  Sum1/1 -> Scope/2, Mux14/2  "Noise x"
  Sum2/1 -> Scope/3, Mux14/3  "Noise y"
  Mux14/1 -> Manual Switch Noise/1
  Mux1/1 -> Gain1/1
  Manual Switch Noise/1 -> Gain/1
  Demux/2 -> Noise_x/1
  Demux/1 -> Noise_theta/1
  Demux/3 -> Noise_y/1
  Sine Wave10/1 -> Sum3/2
  Sine Wave9/1 -> Sum3/1
  Sine Wave11/1 -> Sum3/3
  Sum3/1 -> Scope/4, Mux14/4  "Noise z"
  Demux/4 -> Noise_z/1
  Constant1/1 -> Mux1/2
  Constant/1 -> Mux1/1
  Constant2/1 -> Mux1/3
  Constant3/1 -> Mux1/4
  Gain/1 -> Demux/1
  Gain1/1 -> Manual Switch Noise/2

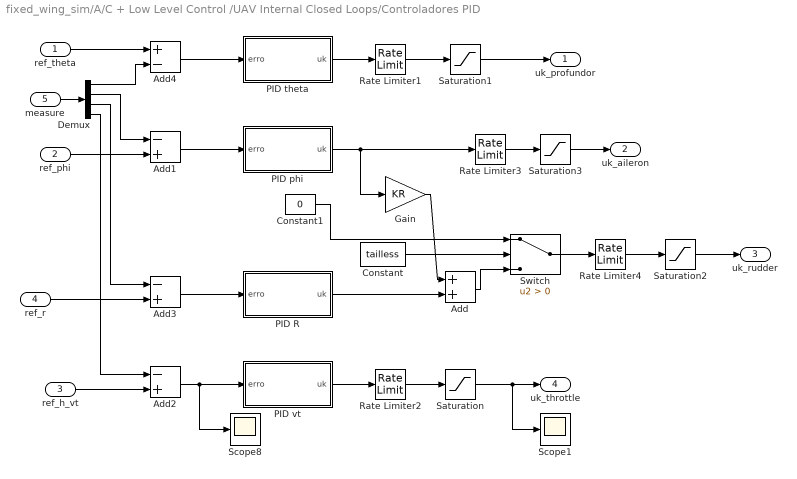
== system fixed_wing_sim/A/C + Low Level Control /UAV Internal Closed Loops/Controladores PID ==
  ref_theta : Inport
  ref_phi : Inport  Port=2
  ref_h_vt : Inport  Port=3
  ref_r : Inport  Port=4
  measure : Inport  Port=5
  Add : Sum
  Add1 : Sum  Inputs=-+
  Add2 : Sum  Inputs=-+
  Add3 : Sum  Inputs=-+
  Add4 : Sum  Inputs=+-
  Constant : Constant  Value=tailless
  Constant1 : Constant  Value=0
  Demux : Demux
  Gain : Gain  Gain=KR
  PID R : Subsystem
  PID phi : Subsystem
  PID theta : Subsystem
  PID vt : Subsystem
  Rate Limiter1 : RateLimiter  RisingSlewLimit=servo_rate  FallingSlewLimit=-servo_rate
  Rate Limiter2 : RateLimiter  RisingSlewLimit=motor_rate  FallingSlewLimit=-motor_rate
  Rate Limiter3 : RateLimiter  RisingSlewLimit=servo_rate  FallingSlewLimit=-servo_rate
  Rate Limiter4 : RateLimiter  RisingSlewLimit=servo_rate  FallingSlewLimit=-servo_rate
  Saturation : Saturate  UpperLimit=1  LowerLimit=motor_min
  Saturation1 : Saturate  UpperLimit=elevator_limits(2)  LowerLimit=elevator_limits(1)
  Saturation2 : Saturate  UpperLimit=rudder_limits(2)  LowerLimit=rudder_limits(1)
  Saturation3 : Saturate  UpperLimit=aileron_limits(2)  LowerLimit=aileron_limits(1)
  Scope1 : Scope
  Scope8 : Scope
  Switch : Switch  Criteria=u2 > Threshold
  uk_profundor : Outport
  uk_aileron : Outport  Port=2
  uk_rudder : Outport  Port=3
  uk_throttle : Outport  Port=4
  wires:
  ref_theta/1 -> Add4/1
  Add4/1 -> PID theta/1(erro)
  measure/1 -> Demux/1
  Demux/1 -> Add4/2
  PID theta/1(uk) -> Rate Limiter1/1
  Rate Limiter1/1 -> Saturation1/1
  PID vt/1(uk) -> Rate Limiter2/1
  Rate Limiter2/1 -> Saturation/1
  Add2/1 -> Scope8/1, PID vt/1(erro)
  PID phi/1(uk) -> Rate Limiter3/1, Gain/1
  Rate Limiter3/1 -> Saturation3/1
  Add1/1 -> PID phi/1(erro)
  ref_phi/1 -> Add1/2
  ref_h_vt/1 -> Add2/2
  Constant/1 -> Switch/2
  Rate Limiter4/1 -> Saturation2/1
  Constant1/1 -> Switch/1
  Demux/2 -> Add1/1
  Demux/3 -> Add3/1
  Demux/4 -> Add2/1
  Add3/1 -> PID R/1(erro)
  Switch/1 -> Rate Limiter4/1
  Add/1 -> Switch/3
  Gain/1 -> Add/1
  PID R/1(uk) -> Add/2
  ref_r/1 -> Add3/2
  Saturation1/1 -> uk_profundor/1
  Saturation3/1 -> uk_aileron/1
  Saturation2/1 -> uk_rudder/1
  Saturation/1 -> Scope1/1, uk_throttle/1

== system fixed_wing_sim/A/C + Low Level Control /UAV Internal Closed Loops/UAV model ==
  control : Inport
  turbulence : Inport  Port=2
  Aerodynamics Equations : Subsystem
      mask Display: image(imread('Figures/aerod.jpg'))
  Atmosphere Model : Subsystem
      mask Display: image(imread('Figures/atmosphere.jpg'))
  Body-Axes 6DOF Equations : Subsystem
      mask Display: image(imread('Figures/forces1.jpg'))
  Constant : Constant  Value=gravity
  Motor Equations : Subsystem
      mask Display: image(imread('Figures/motor_G26.jpg'))
  Output : Subsystem
  Scope2 : Scope
  Servos : Subsystem
      mask Display: image(imread('Figures/servo1.jpg'))
  To Workspace3 : ToWorkspace  VariableName=comando_motor  SaveFormat=Structure With Time  SampleTime=-1
  rpm : Terminator
  output_model : Outport
  wires:
  Body-Axes 6DOF Equations/1(var_states) -> Output/1(states), Aerodynamics Equations/1(var_states), Atmosphere Model/1(var_states)
  Aerodynamics Equations/1(F_Aero_ABC) -> Body-Axes 6DOF Equations/1(F_Aero_ABC)  "Fa_ABC"
  Servos/1(angle_servos) -> Aerodynamics Equations/3(servos)  "command_servos"
  Body-Axes 6DOF Equations/2(acc_x_y_z) -> Output/2(acc)  "acc"
  Aerodynamics Equations/4(V_wind) -> Output/3(V_WIND), Motor Equations/1(Airspeed)  "V_WIND"
  Output/1(Out_model) -> output_model/1
  Constant/1 -> Atmosphere Model/2(gravity)
  Atmosphere Model/1(atmosphere) -> Aerodynamics Equations/2(atmosphere), Motor Equations/2(Atmosphere)
  Aerodynamics Equations/3(F_Tail_ABC) -> Body-Axes 6DOF Equations/3(F_tail_ABC)  "F_tail_ABC"
  Motor Equations/1(F_Thrust_ABC) -> Body-Axes 6DOF Equations/4(F_Thrust_ABC)  "F_Thrust"
  Aerodynamics Equations/2(M_Aero_ABC) -> Body-Axes 6DOF Equations/2(M_Aero_ABC)  "Ma_ABC"
  Servos/2(th_servo) -> Scope2/1, To Workspace3/1, Motor Equations/3(throttle)  "throttle 0% a 100%"
  Motor Equations/2(Delta_V_EH) -> Aerodynamics Equations/4(Delta_V_EH)  "Delta_V_EH"
  turbulence/1 -> Body-Axes 6DOF Equations/5(turb_NED)
  control/1 -> Servos/1(control)
  Body-Axes 6DOF Equations/3(v_ABC') -> Aerodynamics Equations/5(v_ABC')
  Body-Axes 6DOF Equations/4(V_NED) -> Output/4(V_NED)
  Motor Equations/3(RPM) -> rpm/1

== system fixed_wing_sim/A/C + Low Level Control /UAV Internal Closed Loops/Controladores PID/PID R ==
  erro : Inport
  Add : Sum  Inputs=+-++
  Constant : Constant  Value=TI_r
  Divide : Product  Inputs=*/
  Gain : Gain  Gain=KC_r
  Gain1 : Gain
  Gain2 : Gain  Gain=1/rho
  Integrator : Integrator  InitialCondition=u0_uav(3)  LimitOutput=on  UpperSaturationLimit=perc_int_max*rudder_limits(2)  LowerSaturationLimit=-perc_int_max*rudder_limits(2)
  Transfer Fcn : TransferFcn  Numerator=[1/rho]  Denominator=[rho*TD_r 1]
  uk : Outport
  wires:
  Add/1 -> uk/1
  Transfer Fcn/1 -> Add/2
  Integrator/1 -> Add/4
  Divide/1 -> Integrator/1
  Constant/1 -> Divide/2
  Gain1/1 -> Add/1
  Gain2/1 -> Add/3
  erro/1 -> Gain/1
  Gain/1 -> Gain1/1, Transfer Fcn/1, Gain2/1, Divide/1

== system fixed_wing_sim/A/C + Low Level Control /UAV Internal Closed Loops/Controladores PID/PID phi ==
  erro : Inport
  Add : Sum  Inputs=+-++
  Constant : Constant  Value=TI_phi
  Divide : Product  Inputs=*/
  Gain : Gain  Gain=KC_phi
  Gain1 : Gain
  Gain2 : Gain  Gain=1/rho
  Integrator : Integrator  InitialCondition=u0_uav(2)  LimitOutput=on  UpperSaturationLimit=perc_int_max*aileron_limits(2)  LowerSaturationLimit=-perc_int_max*aileron_limits(2)
  Transfer Fcn : TransferFcn  Numerator=[1/rho]  Denominator=[rho*TD_phi 1]
  uk : Outport
  wires:
  Add/1 -> uk/1
  Transfer Fcn/1 -> Add/2
  Integrator/1 -> Add/4
  Divide/1 -> Integrator/1
  Constant/1 -> Divide/2
  Gain1/1 -> Add/1
  Gain2/1 -> Add/3
  erro/1 -> Gain/1
  Gain/1 -> Gain1/1, Transfer Fcn/1, Gain2/1, Divide/1

== system fixed_wing_sim/A/C + Low Level Control /UAV Internal Closed Loops/Controladores PID/PID theta ==
  erro : Inport
  Add : Sum  Inputs=+-++
  Constant : Constant  Value=TI_theta
  Divide : Product  Inputs=*/
  Gain : Gain  Gain=KC_theta
  Gain1 : Gain
  Gain2 : Gain  Gain=1/rho
  Integrator : Integrator  InitialCondition=u0_uav(1)  LimitOutput=on  UpperSaturationLimit=perc_int_max*elevator_limits(2)  LowerSaturationLimit=-perc_int_max*elevator_limits(2)
  Transfer Fcn : TransferFcn  Numerator=[1/rho]  Denominator=[rho*TD_theta 1]
  uk : Outport
  wires:
  Add/1 -> uk/1
  Transfer Fcn/1 -> Add/2
  Integrator/1 -> Add/4
  Divide/1 -> Integrator/1
  Constant/1 -> Divide/2
  Gain1/1 -> Add/1
  Gain2/1 -> Add/3
  erro/1 -> Gain/1
  Gain/1 -> Gain1/1, Transfer Fcn/1, Gain2/1, Divide/1

== system fixed_wing_sim/A/C + Low Level Control /UAV Internal Closed Loops/Controladores PID/PID vt ==
  erro : Inport
  Abs : Abs
  Add : Sum
  Constant : Constant  Value=TI_vt
  Divide : Product  Inputs=*/
  Gain : Gain
  Gain2 : Gain  Gain=KC_vt
  Integrator : Integrator  InitialCondition=u0_uav(4)  LimitOutput=on  UpperSaturationLimit=1 - motor_min  LowerSaturationLimit=2*motor_min
  Scope3 : Scope
  Scope8 : Scope
  Switch : Switch  Criteria=u2 > Threshold  Threshold=1e-2
  uk : Outport
  wires:
  Add/1 -> Scope3/1, uk/1
  erro/1 -> Abs/1, Gain2/1
  Gain2/1 -> Divide/1, Gain/1
  Constant/1 -> Divide/2
  Gain/1 -> Add/1
  Abs/1 -> Switch/2
  Integrator/1 -> Add/2, Scope8/1
  Divide/1 -> Integrator/1

== system fixed_wing_sim/A/C + Low Level Control /UAV Internal Closed Loops/UAV model/Aerodynamics Equations ==
  var_states : Inport
  atmosphere : Inport  Port=2
  servos : Inport  Port=3
  Delta_V_EH : Inport  Port=4
  v_ABC' : Inport  Port=5
  Bus Creator1 : BusCreator  Inputs=3
  Bus Creator2 : BusCreator  Inputs=3
  Bus Selector1 : BusSelector  OutputSignals=P,Q,R
  Bus Selector2 : BusSelector  OutputSignals=density (Kg/m3)
  Demux : Demux  Outputs=3
  F_Aero_WIND : Subsystem
  F_TAIL_WIND --> F_ABC : Subsystem
  F_Tail_WIND : Subsystem
  F_WIND --> F_ABC : Subsystem
  M_Aero_WIND : Subsystem
  U' V' W' --> VT,alpha,beta : Subsystem
  "U' V' W' --> Vtail, alpha_t" : Subsystem
  F_Aero_ABC : Outport
  M_Aero_ABC : Outport  Port=2
  F_Tail_ABC : Outport  Port=3
  V_wind : Outport  Port=4
  wires:
  var_states/1 -> Bus Selector1/1
  Bus Selector1/1 -> Bus Creator1/1  "<P>"
  Bus Selector1/2 -> Bus Creator1/2  "<Q>"
  Bus Selector1/3 -> Bus Creator1/3  "<R>"
  M_Aero_WIND/1(M_ABC) -> M_Aero_ABC/1
  Bus Creator1/1 -> F_Aero_WIND/4(w_ABC), M_Aero_WIND/4(w_ABC), "U' V' W' --> Vtail, alpha_t"/2(w_ABC)
  servos/1 -> F_Aero_WIND/2(servos), M_Aero_WIND/2(servos), F_Tail_WIND/2(servos)
  atmosphere/1 -> Bus Selector2/1
  F_WIND --> F_ABC/1(ABC) -> F_Aero_ABC/1
  F_Aero_WIND/1(F_WIND) -> F_WIND --> F_ABC/2(WIND)
  Bus Selector2/1 -> M_Aero_WIND/3(density), F_Aero_WIND/3(density), F_Tail_WIND/3(density)  "<density (Kg/m3)>"
  U' V' W' --> VT,alpha,beta/1(v_WIND) -> V_wind/1, F_Aero_WIND/1(v_WIND), M_Aero_WIND/1(v_WIND), "U' V' W' --> Vtail, alpha_t"/3(wind), F_Tail_WIND/5(teste_V), F_WIND --> F_ABC/1(v_WIND)
  "U' V' W' --> Vtail, alpha_t"/1(v_TAIL) -> F_Tail_WIND/1(v_WIND), F_TAIL_WIND --> F_ABC/1(v_WIND)
  F_TAIL_WIND --> F_ABC/1(ABC) -> F_Tail_ABC/1
  F_Tail_WIND/1(F_Tail_WIND) -> F_TAIL_WIND --> F_ABC/2(WIND)
  Delta_V_EH/1 -> F_Tail_WIND/4(Delta_V_EH)
  Bus Creator2/1 -> U' V' W' --> VT,alpha,beta/1(v_ABC), "U' V' W' --> Vtail, alpha_t"/1(v_ABC)
  Demux/1 -> Bus Creator2/1  "U"
  Demux/2 -> Bus Creator2/2  "V"
  Demux/3 -> Bus Creator2/3  "W"
  v_ABC'/1 -> Demux/1

== system fixed_wing_sim/A/C + Low Level Control /UAV Internal Closed Loops/UAV model/Atmosphere Model ==
  var_states : Inport
  gravity : Inport  Port=2
  Bus Creator : BusCreator  Inputs=4
  Standard Atmosphere : Subsystem
  atmosphere : Outport
  wires:
  var_states/1 -> Standard Atmosphere/1(var_states)
  gravity/1 -> Standard Atmosphere/2(g)
  Bus Creator/1 -> atmosphere/1
  Standard Atmosphere/1(rho (kg/m3)) -> Bus Creator/1
  Standard Atmosphere/2(a (m/s)) -> Bus Creator/2
  Standard Atmosphere/3(T (K)) -> Bus Creator/3
  Standard Atmosphere/4(P (N/m2)) -> Bus Creator/4

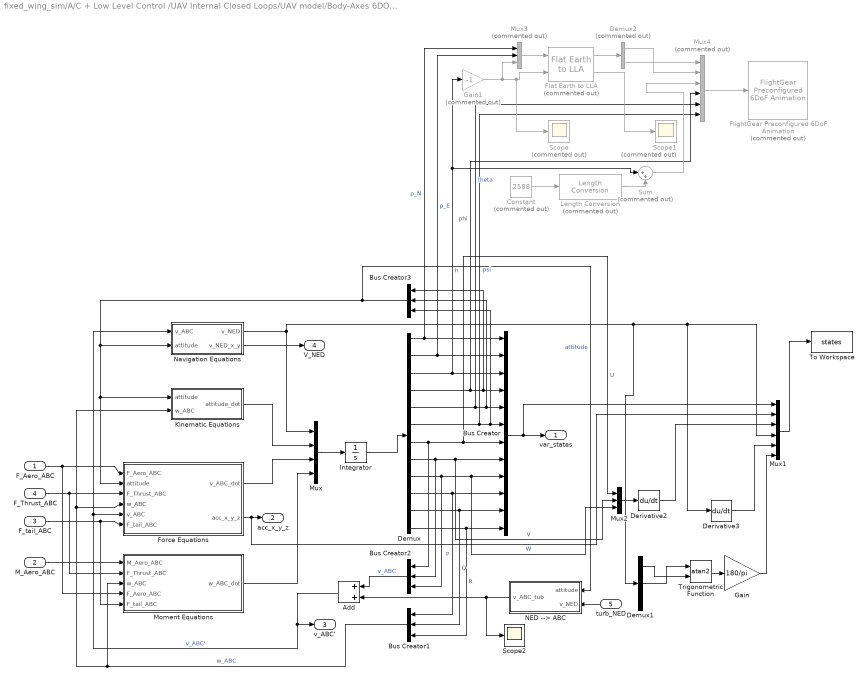
== system fixed_wing_sim/A/C + Low Level Control /UAV Internal Closed Loops/UAV model/Body-Axes 6DOF Equations ==
  F_Aero_ABC : Inport
  M_Aero_ABC : Inport  Port=2
  F_tail_ABC : Inport  Port=3
  F_Thrust_ABC : Inport  Port=4
  turb_NED : Inport  Port=5
  Add : Sum
  Bus Creator : BusCreator  Inputs=12
  Bus Creator1 : BusCreator  Inputs=3
  Bus Creator2 : BusCreator  Inputs=3
  Bus Creator3 : BusCreator  Inputs=3
  Constant : Constant  Commented=on  Value=2588
  Demux : Demux  Outputs=12
  Demux1 : Demux  Outputs=3
  Demux2 : Demux  Commented=on  Outputs=2
  Derivative2 : Derivative
  Derivative3 : Derivative
  Flat Earth to LLA : aerolibtransform2/Flat Earth to LLA  Commented=on  units=Metric (MKS)  ptype=Earth (WGS84)  F=1/298.257223563  R=6378137  LL0=[-19.869928 -43.962819]  psi=0
  FlightGear Preconfigured 6DoF Animation : aerolibfltsims/FlightGear Preconfigured 6DoF Animation  Commented=on  xFlightGearVersion=v2.12  DestinationIpAddress=127.0.0.1  DestinationPort=5502  SampleTime=ts_sim
  Force Equations : Subsystem
  Gain : Gain  Gain=180/pi
  Gain1 : Gain  Commented=on  Gain=-1
  Integrator : Integrator  InitialCondition=x0_uav
  Kinematic Equations : Subsystem
  Length Conversion : aerolibconvert2/Length Conversion  Commented=on  IU=ft  OU=m
  Moment Equations : Subsystem
  Mux : Mux
  Mux1 : Mux  Inputs=6
  Mux2 : Mux  Inputs=3
  Mux3 : Mux  Commented=on  Inputs=3
  Mux4 : Mux  Commented=on  Inputs=6
  NED --> ABC : Subsystem
  Navigation Equations : Subsystem
  Scope : Scope  Commented=on
  Scope1 : Scope  Commented=on
  Scope2 : Scope
  Sum : Sum  Commented=on  Inputs=|++
  To Workspace : ToWorkspace  VariableName=states  SaveFormat=Structure With Time  SampleTime=-1
  Trigonometric Function : Trigonometry  Operator=atan2
  var_states : Outport
  acc_x_y_z : Outport  Port=2
  v_ABC' : Outport  Port=3
  V_NED : Outport  Port=4
  wires:
  Navigation Equations/1(v_NED) -> Demux1/1, Derivative3/1, Mux1/4, Mux/1
  Kinematic Equations/1(attitude_dot) -> Mux/2
  Force Equations/1(v_ABC_dot) -> Mux/3
  Mux/1 -> Integrator/1
  Integrator/1 -> Demux/1
  Demux/1 -> Mux3/1, Bus Creator/1  "p_N"
  Demux/2 -> Mux3/2, Bus Creator/2  "p_E"
  Demux/7 -> Mux2/1, Bus Creator/7, Bus Creator2/1  "U"
  Demux/8 -> Mux2/2, Bus Creator/8, Bus Creator2/2  "V"
  Demux/9 -> Mux2/3, Bus Creator/9, Bus Creator2/3  "W"
  Demux/10 -> Bus Creator1/1, Bus Creator/10  "P"
  Demux/11 -> Bus Creator/11, Bus Creator1/2  "Q"
  Demux/12 -> Bus Creator/12, Bus Creator1/3  "R"
  F_Thrust_ABC/1 -> Force Equations/3(F_Thrust_ABC), Moment Equations/2(F_Thrust_ABC)
  F_Aero_ABC/1 -> Force Equations/1(F_Aero_ABC), Moment Equations/4(F_Aero_ABC)
  Bus Creator1/1 -> Force Equations/4(w_ABC), Kinematic Equations/2(w_ABC), Moment Equations/3(w_ABC)  "w_ABC"
  Bus Creator3/1 -> Navigation Equations/2(attitude), Force Equations/2(attitude), Kinematic Equations/1(attitude), NED --> ABC/1(attitude)  "attitude"
  Moment Equations/1(w_ABC_dot) -> Mux/4
  M_Aero_ABC/1 -> Moment Equations/1(M_Aero_ABC)
  Force Equations/2(acc_x_y_z) -> Mux1/2, acc_x_y_z/1
  F_tail_ABC/1 -> Force Equations/6(F_tail_ABC), Moment Equations/5(F_tail_ABC)
  Demux/6 -> Mux4/6, Bus Creator/6, Bus Creator3/3  "psi"
  Demux/4 -> Mux4/4, Bus Creator/4, Bus Creator3/1  "phi"
  Demux/5 -> Mux4/5, Bus Creator/5, Bus Creator3/2  "theta"
  Bus Creator/1 -> Mux1/1, var_states/1
  turb_NED/1 -> NED --> ABC/2(v_NED)
  Bus Creator2/1 -> Add/1  "v_ABC"
  NED --> ABC/1(v_ABC_tub) -> Scope2/1, Add/2
  Add/1 -> Force Equations/5(v_ABC), Navigation Equations/1(v_ABC), v_ABC'/1  "v_ABC'"
  Navigation Equations/2(v_NED_x_y) -> V_NED/1
  Demux/3 -> Gain1/1, Sum/1, Bus Creator/3  "h"
  Mux1/1 -> To Workspace/1
  Mux2/1 -> Derivative2/1
  Derivative2/1 -> Mux1/3
  Derivative3/1 -> Mux1/5
  Trigonometric Function/1 -> Gain/1
  Gain/1 -> Mux1/6
  Demux1/2 -> Trigonometric Function/1
  Demux1/1 -> Trigonometric Function/2
  Mux3/1 -> Flat Earth to LLA/1
  Flat Earth to LLA/1 -> Demux2/1
  Demux2/1 -> Mux4/2
  Demux2/2 -> Mux4/1
  Mux4/1 -> FlightGear Preconfigured 6DoF Animation/1
  Flat Earth to LLA/2 -> Scope1/1
  Sum/1 -> Mux4/3
  Constant/1 -> Length Conversion/1
  Length Conversion/1 -> Sum/2
  Gain1/1 -> Mux3/3, Scope/1, Flat Earth to LLA/2

== system fixed_wing_sim/A/C + Low Level Control /UAV Internal Closed Loops/UAV model/Motor Equations ==
  Airspeed : Inport
  Atmosphere : Inport  Port=2
  throttle : Inport  Port=3
  Bus Selector1 : BusSelector  OutputSignals=density (Kg/m3)
  Bus Selector4 : BusSelector  OutputSignals=VT
  C_T : Lookup_n-D  BreakpointsForDimension1=V_save  BreakpointsForDimension2=throthle_save  Table=CT_save(:,:)  InputSameDT=on
  Constant : Constant  Value=F_T
  Constant1 : Constant  Value=simple_motor_model
  Constant2 : Constant  Value=2
  Constant3 : Constant  Value=4
  Constant4 : Constant  Value=D_hel
  Constant5 : Constant  Value=0
  Gain1 : Gain  Gain=1/60
  J : Lookup_n-D  BreakpointsForDimension1=V_save  BreakpointsForDimension2=throthle_save  Table=J_save(:,:)  InputSameDT=on
  Lookup Table : Lookup  InputValues=Delta_V_J  Table=Delta_V_EH
  Math Function : Math  Operator=pow  SaturateOnIntegerOverflow=on
  Math Function1 : Math  Operator=pow  SaturateOnIntegerOverflow=on
  Mux : Mux  Inputs=3
  Product : Product  RndMeth=Zero
  Product1 : Product  Inputs=****  RndMeth=Zero
  RPM (Omega) : Lookup_n-D  BreakpointsForDimension1=V_save  BreakpointsForDimension2=throthle_save  Table=rpm_save(:,:)  InputSameDT=on
  Switch : Switch  Criteria=u2 > Threshold  Threshold=0.5
  uncertain RPM1 : Gain  Gain=delta_FT
  F_Thrust_ABC : Outport
  Delta_V_EH : Outport  Port=2
  RPM : Outport  Port=3
  wires:
  Constant/1 -> Product/1
  Airspeed/1 -> Bus Selector4/1
  Bus Selector4/1 -> J/1, RPM (Omega)/1, C_T/1  "<VT>"
  C_T/1 -> Product1/1
  throttle/1 -> C_T/2, J/2, RPM (Omega)/2, Product/2
  RPM (Omega)/1 -> Gain1/1, RPM/1
  Constant2/1 -> Math Function/2
  Constant4/1 -> Math Function1/1
  Constant3/1 -> Math Function1/2
  Math Function/1 -> Product1/2
  Math Function1/1 -> Product1/3
  Gain1/1 -> Math Function/1  "rot/s"
  J/1 -> Lookup Table/1
  Lookup Table/1 -> Delta_V_EH/1
  Mux/1 -> F_Thrust_ABC/1
  Constant5/1 -> Mux/2, Mux/3
  uncertain RPM1/1 -> Mux/1
  Product1/1 -> Switch/3
  Switch/1 -> uncertain RPM1/1
  Constant1/1 -> Switch/2
  Product/1 -> Switch/1
  Atmosphere/1 -> Bus Selector1/1
  Bus Selector1/1 -> Product1/4  "<density (Kg/m3)>"
